simulink model "Design_of_an_Energy_Efficient_Hybrid_Electric_Vehicle"  (R2023a)
settings: Solver=FixedStepDiscrete  StartTime=0  StopTime=110  RelTol=1e-3  EnableMultiTasking=on
PreLoadFcn:
  | power_motordrive_IPMSM_FOC_data
InitFcn:
  | power_motordrive_IPMSM_FOC_data
  | Cdc  = 0.001;      % DC-link capacitor  [F]
  | AH0  = 280;        % Initial battery charge [hr*A]
  | Tmax=410;
  | 
  | %% Vehicle Parameters for Vehicle Dynamics 2
  | vehicle_mass = 2111;
  | wheel_radius = 0.228;
  | area =2.22;
  | drag_coefficient = 0.23;
  | air_density = 1.204;
  | gravity = 9.81;
  | rolling_res_ratio = 0.02;
  | 
  | % Differential drive parameters
  | gear_ratio = 5;
  | i_t   = gear_ratio ;
  | Rw=wheel_radius;
  | 
  | 
  | %% Sliding Mode Observer
  | pmsm.N_max=wmax;
  | pmsm.p=p
  | pmsm.Ld=Ld;
  | pmsm.Lq=Lq;
  | pmsm.Rs=Rs;
  | PU_System.V_base=(Vdc_nom/sqrt(3));
  | PU_System.I_base=lambda/(Lq-Ld);
  | max_torque=400
  | force_max_pedal=500
  | braking_torque_to_pedal_force_ratio=-4
undefined symbols (not defined in the file): BlkSampleTime, CurrentObserverGain, dataType, DiscIntNeverNeededParam, Fsw, gcbh, Ki_Ireg, Ki_wreg, Kp_Ireg, Kp_wreg, L_smo_gain, lambda, Ld, Limit_Ireg, Limit_wreg, Lq, MaxApplicationSpeed, MaxStatorCurrent, MaxStatorVoltage, NumBits1, NumBits2, p, Pmsm, PolePairs, QPLL, rpm_data, Sensorless, sigbuilder_block, SlidingLimit, Slope1, Slope2, sps_rtmsupport, StatorInductance, StatorResistance, Tmax_data, Tnom, Ts, Vdc_nom, wmax
libraries: fl_lib x27, nesl_utility x24, simulink x23, mcbcontrolslib x15, fl_ps_legacy_lib x9, spsStairGeneratorLib x7, sdl_lib x6, ee_lib x4, mcbpositiondecoderlib x4, BoomBox x3, tiiqmathlib x2, autolibshared x2
(part 3 of 4)

== system Design_of_an_Energy_Efficient_Hybrid_Electric_Vehicle/FOC/Speed Regulator1/PI regulator with anti-windup D1 ==
  note: Anti-windup mechanism: Method of conditionnal integration
      |
      | The integration is suspended if saturation occurs and the
      | control error is of the same sign as the control signal.
      |
      | [1] L.Rundqwist, "Anti-Reset Windup for PID Controllers," Ph.D. Thesis TRFT-1033,
      | Departement of Automatic Control, Lund Institute of Technology, Lund, Sweeden, 1991.
  Error : Inport  SampleTime=Ts
  Compare To Zero : simulink/Logic and Bit Operations/Compare To Zero  relop=>  OutDataTypeStr=uint8  ZeroCross=off
  Compare To Zero1 : simulink/Logic and Bit Operations/Compare To Zero  relop=<  OutDataTypeStr=uint8  ZeroCross=off
  Constant : Constant  Value=0
  Constant1 : Constant  Value=UpperLimit
  Constant3 : Constant  Value=LowerLimit
  Discrete-Time Integrator : DiscreteIntegrator  IntegratorMethod=Integration: Trapezoidal  InitialCondition=Init  SampleTime=Ts  LimitOutput=on  UpperSaturationLimit=UpperLimit  LowerSaturationLimit=LowerLimit  ShowStatePort=on  ICPrevOutput=DiscIntNeverNeededParam  ICPrevScaledInput=DiscIntNeverNeededParam
  Kp4 : Gain  Gain=Kp  SaturateOnIntegerOverflow=on  SampleTime=Ts  OutDataTypeStr=Inherit: Same as input  ParamDataTypeStr=Inherit: Same as input
  Kp5 : Gain  Gain=Ki  SaturateOnIntegerOverflow=on  SampleTime=Ts  OutDataTypeStr=Inherit: Same as input  ParamDataTypeStr=Inherit: Same as input
  Logical Operator : Logic  AllPortsSameDT=off  OutDataTypeStr=boolean
  Logical Operator1 : Logic  AllPortsSameDT=off  OutDataTypeStr=boolean
  Logical Operator2 : Logic  Operator=OR  AllPortsSameDT=off  OutDataTypeStr=boolean
  Relational Operator : RelationalOperator  OutDataTypeStr=boolean  InputSameDT=off
  Relational Operator1 : RelationalOperator  Operator=<=  OutDataTypeStr=boolean  InputSameDT=off
  Saturation2 : Saturate  UpperLimit=UpperLimit  LowerLimit=LowerLimit  SampleTime=Ts
  Sum1 : Sum  InputSameDT=on  SaturateOnIntegerOverflow=on  SampleTime=Ts  OutDataTypeStr=Inherit: Same as first input
  Sum6 : Sum  InputSameDT=on  SaturateOnIntegerOverflow=on  SampleTime=Ts  OutDataTypeStr=Inherit: Same as first input
  Switch : Switch  Criteria=u2 > Threshold  SaturateOnIntegerOverflow=off  InputSameDT=off
  Zero-Order Hold : ZeroOrderHold  SampleTime=Ts
  Out : Outport  SampleTime=Ts  InitialOutput=0
  wires:
  Constant/1 -> Switch/1
  Zero-Order Hold/1 -> Sum1/2, Sum6/1
  Discrete-Time Integrator/State -> Sum1/1
  Sum1/1 -> Relational Operator1/1, Relational Operator/1
  Logical Operator2/1 -> Switch/2
  Relational Operator/1 -> Logical Operator/1  "UpperLimit_is_Reached"
  Relational Operator1/1 -> Logical Operator1/1  "LowerLimit_Is_Reached"
  Constant1/1 -> Relational Operator/2
  Constant3/1 -> Relational Operator1/2
  Compare To Zero/1 -> Logical Operator/2  "Error_is_positive"
  Logical Operator/1 -> Logical Operator2/1
  Logical Operator1/1 -> Logical Operator2/2
  Compare To Zero1/1 -> Logical Operator1/2  "Error_is_negative"
  Error/1 -> Compare To Zero1/1, Compare To Zero/1, Kp4/1, Kp5/1
  Sum6/1 -> Saturation2/1
  Kp4/1 -> Zero-Order Hold/1
  Discrete-Time Integrator/1 -> Sum6/2
  Saturation2/1 -> Out/1
  Switch/1 -> Discrete-Time Integrator/1
  Kp5/1 -> Switch/3

== system Design_of_an_Energy_Efficient_Hybrid_Electric_Vehicle/FOC/Speed Regulator1/PI regulator with anti-windup D2 ==
  note: Anti-windup mechanism: Method of conditionnal integration
      |
      | The integration is suspended if saturation occurs and the
      | control error is of the same sign as the control signal.
      |
      | [1] L.Rundqwist, "Anti-Reset Windup for PID Controllers," Ph.D. Thesis TRFT-1033,
      | Departement of Automatic Control, Lund Institute of Technology, Lund, Sweeden, 1991.
  Error : Inport  SampleTime=Ts
  Compare To Zero : simulink/Logic and Bit Operations/Compare To Zero  relop=>  OutDataTypeStr=uint8  ZeroCross=off
  Compare To Zero1 : simulink/Logic and Bit Operations/Compare To Zero  relop=<  OutDataTypeStr=uint8  ZeroCross=off
  Constant : Constant  Value=0
  Constant1 : Constant  Value=UpperLimit
  Constant3 : Constant  Value=LowerLimit
  Discrete-Time Integrator : DiscreteIntegrator  IntegratorMethod=Integration: Trapezoidal  InitialCondition=Init  SampleTime=Ts  LimitOutput=on  UpperSaturationLimit=UpperLimit  LowerSaturationLimit=LowerLimit  ShowStatePort=on  ICPrevOutput=DiscIntNeverNeededParam  ICPrevScaledInput=DiscIntNeverNeededParam
  Kp4 : Gain  Gain=Kp  SaturateOnIntegerOverflow=on  SampleTime=Ts  OutDataTypeStr=Inherit: Same as input  ParamDataTypeStr=Inherit: Same as input
  Kp5 : Gain  Gain=Ki  SaturateOnIntegerOverflow=on  SampleTime=Ts  OutDataTypeStr=Inherit: Same as input  ParamDataTypeStr=Inherit: Same as input
  Logical Operator : Logic  AllPortsSameDT=off  OutDataTypeStr=boolean
  Logical Operator1 : Logic  AllPortsSameDT=off  OutDataTypeStr=boolean
  Logical Operator2 : Logic  Operator=OR  AllPortsSameDT=off  OutDataTypeStr=boolean
  Relational Operator : RelationalOperator  OutDataTypeStr=boolean  InputSameDT=off
  Relational Operator1 : RelationalOperator  Operator=<=  OutDataTypeStr=boolean  InputSameDT=off
  Saturation2 : Saturate  UpperLimit=UpperLimit  LowerLimit=LowerLimit  SampleTime=Ts
  Sum1 : Sum  InputSameDT=on  SaturateOnIntegerOverflow=on  SampleTime=Ts  OutDataTypeStr=Inherit: Same as first input
  Sum6 : Sum  InputSameDT=on  SaturateOnIntegerOverflow=on  SampleTime=Ts  OutDataTypeStr=Inherit: Same as first input
  Switch : Switch  Criteria=u2 > Threshold  SaturateOnIntegerOverflow=off  InputSameDT=off
  Zero-Order Hold : ZeroOrderHold  SampleTime=Ts
  Out : Outport  SampleTime=Ts  InitialOutput=0
  wires:
  Kp5/1 -> Switch/3
  Switch/1 -> Discrete-Time Integrator/1
  Saturation2/1 -> Out/1
  Discrete-Time Integrator/1 -> Sum6/2
  Kp4/1 -> Zero-Order Hold/1
  Sum6/1 -> Saturation2/1
  Error/1 -> Kp5/1, Kp4/1, Compare To Zero/1, Compare To Zero1/1
  Compare To Zero1/1 -> Logical Operator1/2  "Error_is_negative"
  Logical Operator1/1 -> Logical Operator2/2
  Logical Operator/1 -> Logical Operator2/1
  Compare To Zero/1 -> Logical Operator/2  "Error_is_positive"
  Constant3/1 -> Relational Operator1/2
  Constant1/1 -> Relational Operator/2
  Relational Operator1/1 -> Logical Operator1/1  "LowerLimit_Is_Reached"
  Relational Operator/1 -> Logical Operator/1  "UpperLimit_is_Reached"
  Logical Operator2/1 -> Switch/2
  Sum1/1 -> Relational Operator/1, Relational Operator1/1
  Discrete-Time Integrator/State -> Sum1/1
  Zero-Order Hold/1 -> Sum6/1, Sum1/2
  Constant/1 -> Switch/1

== system Design_of_an_Energy_Efficient_Hybrid_Electric_Vehicle/FOC/Speed Regulator1/VdVq Limiter ==
  VdVq_unsat : Inport
  Complex to Magnitude-Angle1 : ComplexToMagnitudeAngle
  Complex to Real-Imag : ComplexToRealImag
  Demux : Demux  Outputs=2
  Hypot : Math  Operator=hypot
  Magnitude-Angle to Complex : MagnitudeAngleToComplex
  Mux : Mux  Inputs=2
  Real-Imag to Complex : RealImagToComplex
  Saturation1 : Saturate  UpperLimit=2/sqrt(3)  LowerLimit=0
  VdVq : Outport
  ModIndex : Outport  Port=2
  wires:
  Real-Imag to Complex/1 -> Complex to Magnitude-Angle1/1
  Saturation1/1 -> Magnitude-Angle to Complex/1
  Complex to Magnitude-Angle1/2 -> Magnitude-Angle to Complex/2
  Complex to Magnitude-Angle1/1 -> Saturation1/1
  Magnitude-Angle to Complex/1 -> Complex to Real-Imag/1
  Demux/1 -> Real-Imag to Complex/1
  Demux/2 -> Real-Imag to Complex/2
  VdVq_unsat/1 -> Demux/1
  Complex to Real-Imag/1 -> Hypot/1, Mux/1
  Complex to Real-Imag/2 -> Hypot/2, Mux/2
  Mux/1 -> VdVq/1
  Hypot/1 -> ModIndex/1

== system Design_of_an_Energy_Efficient_Hybrid_Electric_Vehicle/Test_Sequences/Test_Sequence/IDC ==
  Demux : Demux  Tag=STV Demux  Outputs=1
      settings: DisplayOption=none
  FromWs : FromWorkspace  Tag=STV FromWs  VariableName=tuvar  SampleTime=Ts
      SigBuilderData=|
      | common.afterFinalStr = 'Extrapolate'
      | common.sampleTime = 'Ts'
      | dataSet.timeRange = [0 130]
      | dataSet.name = 'Test 1'
      | sbobj.Groups.Name = 'Test 1'
      | sbobj.Groups.Signals.Name = 'Speed'
      | sbobj.Groups.Signals.XData = [0 17 20 28 30 35 40 50 55 60 75 80 90 120 130]
      | sbobj.Groups.Signals.YData = [0 0 17.5 6 6 30 24 24 41 35.5 35.5 31 40 5 -8.4]
      | sbobj.Groups.TimeRange = [0 130]
  Speed : Outport  Tag=STV Outport  VectorParamsAs1DForOutWhenUnconnected=off
  wires:
  FromWs/1 -> Demux/1
  Demux/1 -> Speed/1

== system Design_of_an_Energy_Efficient_Hybrid_Electric_Vehicle/Test_Sequences/Test_Sequence/Load_Torque ==
  Demux : Demux  Tag=STV Demux  Outputs=1
      settings: DisplayOption=none
  FromWs : FromWorkspace  Tag=STV FromWs  VariableName=tuvar
      SigBuilderData=|
      | common.afterFinalStr = 'Extrapolate'
      | common.sampleTime = '0'
      | dataSet.timeRange = [0 14]
      | dataSet.name = 'Test 1'
      | sbobj.Groups.Name = 'Test 1'
      | sbobj.Groups.Signals.Name = 'Signal 2'
      | sbobj.Groups.Signals.XData = [0 4 5 5 14]
      | sbobj.Groups.Signals.YData = [0.945 0.945 0.945 0.3 0.3]
      | sbobj.Groups.TimeRange = [0 14]
  Signal 2 : Outport  Tag=STV Outport
  wires:
  FromWs/1 -> Demux/1
  Demux/1 -> Signal 2/1

== system Design_of_an_Energy_Efficient_Hybrid_Electric_Vehicle/Test_Sequences/Test_Sequence/Ref_Speed ==
  Demux : Demux  Tag=STV Demux  Outputs=1
      settings: DisplayOption=none
  FromWs : FromWorkspace  Tag=STV FromWs  VariableName=tuvar
      SigBuilderData=|
      | common.afterFinalStr = 'Extrapolate'
      | common.sampleTime = '0'
      | dataSet.timeRange = [0 13]
      | dataSet.name = 'Test 1'
      | sbobj.Groups.Name = 'Test 1'
      | sbobj.Groups.Signals.Name = 'Speed'
      | sbobj.Groups.Signals.XData = [0 0.65 1.3 2 4 6 7.5 9.3 12 13]
      | sbobj.Groups.Signals.YData = [0 0 0.2 0.2 1 1 1.5 1.5 0 0]
      | sbobj.Groups.TimeRange = [0 13]
  Speed : Outport  Tag=STV Outport  VectorParamsAs1DForOutWhenUnconnected=off
  wires:
  FromWs/1 -> Demux/1
  Demux/1 -> Speed/1

== system Design_of_an_Energy_Efficient_Hybrid_Electric_Vehicle/FOC/Speed Regulator1/Calculate position and speed/Sliding Mode Observer ==
  InputSignals : Inport
  Data Type Conversion : DataTypeConversion  OutDataTypeStr=boolean  SaturateOnIntegerOverflow=off  RndMeth=Floor
  Demux1 : Demux
  EEMF Model : Subsystem
  Logical Operator : Logic  Operator=NOT  IconShape=distinctive  AllPortsSameDT=off  OutDataTypeStr=boolean
  Mux : Mux  Inputs=2
  Scope : Scope  NumInputPorts=2
  Scope1 : Scope  NumInputPorts=4
  Sliding Mode Observer : Subsystem  Commented=on  mask(Sliding Mode Observer){CurrentObserverGain=.1, SlidingLimit=3, PositionUnit=Per unit, PositionDataType=dataType, SpeedUnit=Per unit, PerUnitSpeed=PU_System.N_base, SpeedDataType=dataType, BlkSampleTime=Ts, StatorResistance=pmsm.Rs, StatorInductance=pmsm.Ld, MaxApplicationSpeed=pmsm.N_max, PolePairs=pmsm.p, MaxStatorVoltage=PU_System.V_base, MaxStatorCurrent=PU_System.I_base}
      mask prompts: CurrentObserverGain "Current observer gain:"; SlidingLimit "Sliding surface limit:"; PositionUnit "Position unit:"; PositionDataType "Position datatype:"; SpeedUnit "Speed unit"; PerUnitSpeed "Per unit speed (RPM):"; SpeedDataType "Speed datatype:"; BlkSampleTime "Block sample time (S):"; StatorResistance "Stator resistance (ohm):"; StatorInductance "Stator inductance (H):"; MaxApplicationSpeed "Maximum application speed (RPM):"; PolePairs "Number of pole pairs:"; MaxStatorVoltage "Per unit reference stator voltage:"; MaxStatorCurrent "Per unit reference stator current:"
      mask help:
      | <p>Compute &#952;<sub>e</sub> (electrical position) and &#969;<sub>m</sub> (mechanical speed) of a PMSM from the measured per unit voltage and current in the stationary reference frame.
      | <br><br>
      | Use the Current observer gain and Sliding surface limit parameters to tune Sliding Mode Observer (SMO). To improve stability, increase the Sliding surface limit or reduce Current observer gain. To reduce distortion, increase the Current observer gain.
      | <br><br>
      | Enter the peak-to-peak line-to-line voltage and peak-to-peak line current of the stator, in the Per unit reference parameters. Ensure that the values for Per Unit reference stator voltage, Per unit reference stator current, and Maximum application speed conform to the maximum applicable limits for the SMO.</P>
      mask init:
      | mcb.internal.SMOCb('MaskInitFcn',gcbh);
      mask Help: eval('mcb.internal.helpview(''slidingmodeobserver'')')
      mask TypeOptions PositionUnit: Degrees | Radians | Per unit
      mask TypeOptions SpeedUnit: Degrees/sec | Radians/sec | RPM | Per unit
      mask Callback SpeedUnit: mcb.internal.SMOCb('SpeedUnit',gcbh);
      mask DialogControl Container4 Prompt: Observer Parameters
      mask DialogControl Container7 Prompt: Motor Parameters
      mask Display:
      | color('black');
      | port_label('input',1, 'V_{\alpha}', 'interpreter', 'tex');
      | port_label('input',2, 'V_{\beta}', 'interpreter', 'tex');
      | port_label('input',3, 'I_{\alpha}', 'interpreter', 'tex');
      | port_label('input',4, 'I_{\beta}', 'interpreter', 'tex');
      | port_label('input',5, 'Rst', 'interpreter', 'tex');
      | port_label('output',1, '\theta_{e}', 'interpreter', 'tex');
      | port_label('output',2, '\omega_{m}', 'interpreter', 'tex');
      | fprintf('SMO');
  Step : Step  SampleTime=0
  Subsystem : Subsystem  Commented=on
  Position/Speed : Outport
  wires:
  Mux/1 -> Position/Speed/1
  Demux1/1 -> EEMF Model/1(Valpha), Scope1/1
  Demux1/2 -> EEMF Model/2(Vbeta), Scope1/2
  Demux1/4 -> EEMF Model/4(Ibeta), Scope1/4  "Ibeta"
  Demux1/3 -> EEMF Model/3(Ialpha), Scope1/3  "Ialpha"
  EEMF Model/1(Theta) -> Scope/1, Mux/1
  EEMF Model/2(Speed) -> Scope/2, Mux/2
  InputSignals/1 -> Demux1/1
  Step/1 -> Data Type Conversion/1
  Logical Operator/1 -> EEMF Model/5(Reset)
  Data Type Conversion/1 -> Logical Operator/1

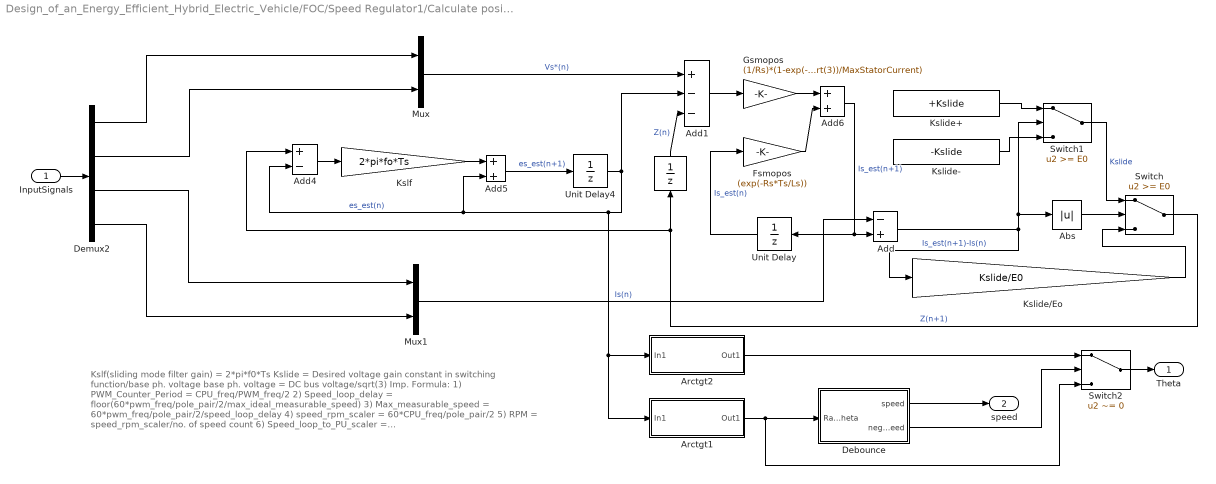
== system Design_of_an_Energy_Efficient_Hybrid_Electric_Vehicle/FOC/Speed Regulator1/Calculate position and speed/Sliding Mode Observer (SMO) ==
  note: Kslf(sliding mode filter gain) = 2*pi*f0*Ts
      | Kslide = Desired voltage gain constant in switching function/base ph. voltage
      | base ph. voltage = DC bus voltage/sqrt(3)
      |
      | Imp. Formula:
      |
      | 1) PWM_Counter_Period = CPU_freq/PWM_freq/2
      | 2) Speed_loop_delay = floor(60*pwm_freq/pole_pair/2/max_ideal_measurable_speed)
      | 3) Max_measurable_speed = 60*pwm_freq/pole_pair/2/speed_loop_delay
      | 4) speed_rpm_scaler = 60*CPU_freq/pole_pair/2
      | 5) RPM = speed_rpm_scaler/no. of speed count
      | 6) Speed_loop_to_PU_scaler = Max_measurable_speed/Speed_per_unit_scaler
      |
      | 7) Fsmopos = exp(-motor.rs/motor.ls/PWM_frequency)
      | 8)Gsmopos = motor.base_voltage/motor.base_current/motor.rs*(1-Fsmopos)
      | 9)motor.base_voltage = 38.29; % Base peak phase voltage (volt), maximum measurable DC Bus(66.32V)/sqrt(3)
      | 10)motor.base_current = 8.6; % Base peak phase current (amp) , maximum measurable peak current
      | 11)motor.base_freq = 200; % Base electrical frequency (Hz)
  InputSignals : Inport
  " " : UnitDelay  SampleTime=-1  HasFrameUpgradeWarning=on
  Abs : Abs  SaturateOnIntegerOverflow=off
  Add : Sum  Inputs=-+  OutDataTypeStr=Inherit: Same as first input
  Add1 : Sum  Inputs=+--  OutDataTypeStr=Inherit: Inherit via back propagation
  Add4 : Sum  Inputs=+-  OutDataTypeStr=Inherit: Same as first input
  Add5 : Sum  OutDataTypeStr=Inherit: Same as first input
  Add6 : Sum  OutDataTypeStr=Inherit: Same as first input
  Arctgt1 : Subsystem
  Arctgt2 : Subsystem
  Debounce : Subsystem
  Demux2 : Demux
  Fsmopos : Gain  Gain=(exp(-Rs*Ts/Ls))  OutDataTypeStr=Inherit: Same as input  ParamDataTypeStr=Inherit: Same as input
  Gsmopos : Gain  Gain=(1/Rs)*(1-exp(-Rs*Ts/Ls)*(MaxStatorVoltage/sqrt(3))/MaxStatorCurrent)  OutDataTypeStr=Inherit: Same as input  ParamDataTypeStr=Inherit: Same as input
  Kslf : Gain  Gain=2*pi*fo*Ts  OutDataTypeStr=Inherit: Same as input  ParamDataTypeStr=Inherit: Same as input
  Kslide+ : Constant  Value=+Kslide  OutDataTypeStr=fixdt(1,32,17)
  Kslide- : Constant  Value=-Kslide  OutDataTypeStr=fixdt(1,32,17)
  Kslide/Eo : Gain  Gain=Kslide/E0  OutDataTypeStr=Inherit: Same as input  ParamDataTypeStr=Inherit: Same as input
  Mux : Mux  Inputs=2
  Mux1 : Mux  Inputs=2
  Switch : Switch  Threshold=E0  OutDataTypeStr=Inherit: Inherit via back propagation  SaturateOnIntegerOverflow=off  InputSameDT=off
  Switch1 : Switch  Threshold=E0  OutDataTypeStr=Inherit: Inherit via back propagation  SaturateOnIntegerOverflow=off  InputSameDT=off
  Switch2 : Switch  Criteria=u2 ~= 0  SaturateOnIntegerOverflow=off  InputSameDT=off
  Unit Delay : UnitDelay  SampleTime=-1  HasFrameUpgradeWarning=on
  Unit Delay4 : UnitDelay  SampleTime=-1  HasFrameUpgradeWarning=on
  Theta : Outport  VectorParamsAs1DForOutWhenUnconnected=off
  speed : Outport  Port=2  VectorParamsAs1DForOutWhenUnconnected=off
  wires:
  Unit Delay/1 -> Fsmopos/1  "Is_est(n)"
  " "/1 -> Add1/3  "Z(n)"
  Add/1 -> Kslide/Eo/1, Abs/1, Switch1/2  "Is_est(n+1)-Is(n)"
  Add1/1 -> Gsmopos/1
  Demux2/2 -> Mux/2
  Mux/1 -> Add1/1  "Vs*(n)"
  Add4/1 -> Kslf/1
  Unit Delay4/1 -> Arctgt2/1(In1), Arctgt1/1(In1), Add5/2, Add4/2, Add1/2  "es_est(n)"
  Kslf/1 -> Add5/1
  Add5/1 -> Unit Delay4/1  "es_est(n+1)"
  Gsmopos/1 -> Add6/1
  Fsmopos/1 -> Add6/2
  Add6/1 -> Add/2, Unit Delay/1  "Is_est(n+1)"
  Demux2/3 -> Mux1/1
  Demux2/4 -> Mux1/2
  Abs/1 -> Switch/2
  Kslide/Eo/1 -> Switch/3
  Switch1/1 -> Switch/1  "Kslide"
  Kslide+/1 -> Switch1/1
  Kslide-/1 -> Switch1/3
  Switch/1 -> Add4/1, " "/1  "Z(n+1)"
  Mux1/1 -> Add/1  "Is(n)"
  Arctgt1/1(Out1) -> Switch2/3, Debounce/1(Raw_theta)
  Arctgt2/1(Out1) -> Switch2/1
  Switch2/1 -> Theta/1
  Debounce/1(speed) -> speed/1
  Debounce/2(negative speed) -> Switch2/2
  InputSignals/1 -> Demux2/1
  Demux2/1 -> Mux/1

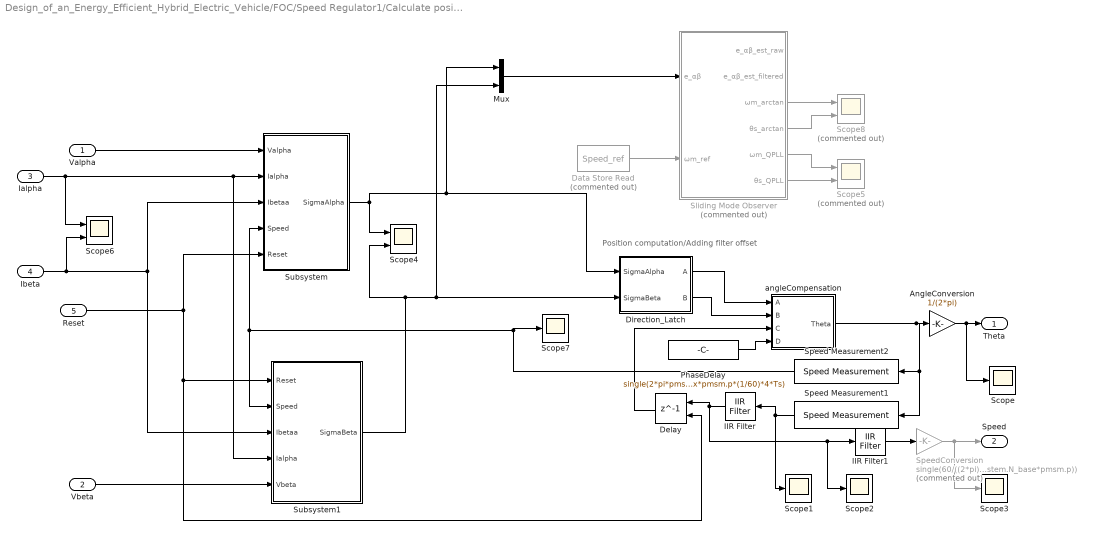
== system Design_of_an_Energy_Efficient_Hybrid_Electric_Vehicle/FOC/Speed Regulator1/Calculate position and speed/Sliding Mode Observer/EEMF Model ==
  note: Position computation/Adding filter offset
  Valpha : Inport
  Vbeta : Inport  Port=2
  Ialpha : Inport  Port=3
  Ibeta : Inport  Port=4
  Reset : Inport  Port=5
  AngleConversion : Gain  Gain=1/(2*pi)  OutDataTypeStr=single
  Data Store Read : DataStoreRead  Commented=on  DataStoreName=Speed_ref  IndexOptions=Index vector (dialog)  Indices=1  OutputSizes=1
  Delay : Delay  DelayLength=1  ExternalReset=Level
      settings: InputPortMap=u0,r5
  Direction_Latch : Subsystem
  IIR Filter : mcbcontrolslib/IIR Filter  VariantControl=Low Pass Filter  VariantSelect=Low-pass  Filter_constant=single(Ts*pmsm.N_max*pmsm.p/120)  advancedSettings=off  Ts=50e-6  cutOff_freq=12.7835
  IIR Filter1 : mcbcontrolslib/IIR Filter  VariantControl=Low Pass Filter  VariantSelect=Low-pass  Filter_constant=single(Ts*pmsm.N_max*pmsm.p/120)  advancedSettings=off  Ts=50e-6  cutOff_freq=12.7835
  Mux : Mux  Inputs=2
  PhaseDelay : Constant  Value=single(2*pi*pmsm.N_max*pmsm.p*(1/60)*4*Ts)  OutDataTypeStr=Inherit: Inherit via back propagation  SampleTime=-1
  Scope{,1..3,7} (5 alike) : Scope
  Scope4 : Scope  NumInputPorts=2
  Scope5 : Scope  Commented=on  NumInputPorts=2
  Scope6 : Scope  NumInputPorts=2
  Scope8 : Scope  Commented=on  NumInputPorts=2
  Sliding Mode Observer : Subsystem  Commented=on
  Speed Measurement1 : mcbpositiondecoderlib/Speed Measurement  PositionUnit=Radians  PositionScalingDatatype=uint32  SpeedCalculationMode=Maximum application speed  SampleTimeAsync=Ts  MaximumApplicationSpeed=pmsm.N_max*pmsm.p  SpeedResolution=5e-6  DelayLength=61  MaximumMeasurableSpeed=24193.5484  MeasurableSpeedResolution=1.1266e-05  SpeedUnit=Radians/Sec  PerUnitSpeed=1000  SpeedDataType=single
  Speed Measurement2 : mcbpositiondecoderlib/Speed Measurement  PositionUnit=Radians  PositionScalingDatatype=uint32  SpeedCalculationMode=Maximum application speed  SampleTimeAsync=Ts  MaximumApplicationSpeed=pmsm.N_max*pmsm.p  SpeedResolution=5e-6  DelayLength=61  MaximumMeasurableSpeed=24193.5484  MeasurableSpeedResolution=1.1266e-05  SpeedUnit=Per unit based on maximum measurable speed  PerUnitSpeed=1000  SpeedDataType=single
  SpeedConversion : Gain  Commented=on  Gain=single(60/((2*pi)*PU_System.N_base*pmsm.p))  OutDataTypeStr=single
  Subsystem : Subsystem
  Subsystem1 : Subsystem
  angleCompensation : Subsystem  TreatAsAtomicUnit=on
  Theta : Outport  VectorParamsAs1DForOutWhenUnconnected=off
  Speed : Outport  Port=2  VectorParamsAs1DForOutWhenUnconnected=off
  wires:
  Reset/1 -> Subsystem/5(Reset), Delay/2, Subsystem1/1(Reset)
  SpeedConversion/1 -> Scope3/1, Speed/1
  Ibeta/1 -> Scope6/2, Subsystem1/3(Ibetaa), Subsystem/3(Ibetaa)
  Vbeta/1 -> Subsystem1/5(Vbeta)
  PhaseDelay/1 -> angleCompensation/4(D)
  Valpha/1 -> Subsystem/1(Valpha)
  angleCompensation/1(Theta) -> Speed Measurement2/1, Speed Measurement1/1, AngleConversion/1
  Speed Measurement1/1 -> Scope1/1, IIR Filter/1
  AngleConversion/1 -> Scope/1, Theta/1
  Direction_Latch/1(A) -> angleCompensation/1(A)
  Ialpha/1 -> Scope6/1, Subsystem1/4(Ialpha), Subsystem/2(Ialpha)
  Direction_Latch/2(B) -> angleCompensation/2(B)
  Delay/1 -> angleCompensation/3(C)
  Subsystem/1(SigmaAlpha) -> Mux/1, Direction_Latch/1(SigmaAlpha), Scope4/1
  Subsystem1/1(SigmaBeta) -> Mux/2, Direction_Latch/2(SigmaBeta), Scope4/2
  IIR Filter/1 -> IIR Filter1/1, Scope2/1, Delay/1
  Speed Measurement2/1 -> Scope7/1, Subsystem/4(Speed), Subsystem1/2(Speed)
  IIR Filter1/1 -> SpeedConversion/1
  Mux/1 -> Sliding Mode Observer/1(e_αβ)
  Data Store Read/1 -> Sliding Mode Observer/2(ωm_ref)
  Sliding Mode Observer/5(ωm_QPLL) -> Scope5/1
  Sliding Mode Observer/6(θs_QPLL) -> Scope5/2
  Sliding Mode Observer/3(ωm_arctan) -> Scope8/1
  Sliding Mode Observer/4(θs_arctan) -> Scope8/2

== system Design_of_an_Energy_Efficient_Hybrid_Electric_Vehicle/FOC/Speed Regulator1/Calculate position and speed/Sliding Mode Observer/Sliding Mode Observer ==
  note: Position computation/Adding filter offset
  Valpha : Inport
  Vbeta : Inport  Port=2
  Ialpha : Inport  Port=3
  Ibeta : Inport  Port=4
  Reset : Inport  Port=5
  AngleConversion : Gain  Gain=1/(2*pi)  OutDataTypeStr=PositionDataType
  Delay : Delay  DelayLength=1  ExternalReset=Level
      settings: InputPortMap=u0,r5
  Direction_Latch : Subsystem
  IIR Filter : mcbcontrolslib/IIR Filter  VariantControl=Low Pass Filter  VariantSelect=Low-pass  Filter_constant=single(BlkSampleTime(1)*MaxApplicationSpeed*PolePairs/120)  advancedSettings=off  Ts=50e-6
  PhaseDelay : Constant  Value=single((StatorResistance+(CurrentObserverGain/SlidingLimit))/StatorInductance)  OutDataTypeStr=Inherit: Inherit via back propagation
  Scope{,1..3} (4 alike) : Scope
  Speed Measurement : mcbpositiondecoderlib/Speed Measurement  PositionUnit=Radians  PositionScalingDatatype=uint32  SpeedCalculationMode=Maximum application speed  SampleTimeAsync=BlkSampleTime  MaximumApplicationSpeed=MaxApplicationSpeed*PolePairs  SpeedResolution=5e-6  DelayLength=14  MaximumMeasurableSpeed=40000  MeasurableSpeedResolution=1.8626e-05  SpeedUnit=Radians/Sec  PerUnitSpeed=1000  SpeedDataType=single
  SpeedConversion : Gain  Gain=single(60/((2*pi)*PerUnitSpeed*PolePairs))  OutDataTypeStr=SpeedDataType
  Subsystem : Subsystem
  Subsystem1 : Subsystem
  angleCompensation : Subsystem  TreatAsAtomicUnit=on
  Theta : Outport  VectorParamsAs1DForOutWhenUnconnected=off
  Speed : Outport  Port=2  VectorParamsAs1DForOutWhenUnconnected=off
  wires:
  Reset/1 -> Delay/2, Subsystem1/3(Reset), Subsystem/3(Reset)
  Subsystem1/1(SigmaBeta) -> Direction_Latch/2(SigmaBeta)
  Subsystem/1(SigmaAlpha) -> Direction_Latch/1(SigmaAlpha)
  Direction_Latch/2(B) -> angleCompensation/2(B)
  Direction_Latch/1(A) -> angleCompensation/1(A)
  AngleConversion/1 -> Theta/1
  Delay/1 -> angleCompensation/3(C)
  PhaseDelay/1 -> angleCompensation/4(D)
  angleCompensation/1(Theta) -> Speed Measurement/1, Scope/1, AngleConversion/1
  Ibeta/1 -> Subsystem1/2(Ibetaa)
  Ialpha/1 -> Subsystem/2(Ialpha)
  Vbeta/1 -> Subsystem1/1(Vbeta)
  Valpha/1 -> Subsystem/1(Valpha)
  Speed Measurement/1 -> Scope1/1, IIR Filter/1
  IIR Filter/1 -> Delay/1, SpeedConversion/1, Scope2/1
  SpeedConversion/1 -> Scope3/1, Speed/1

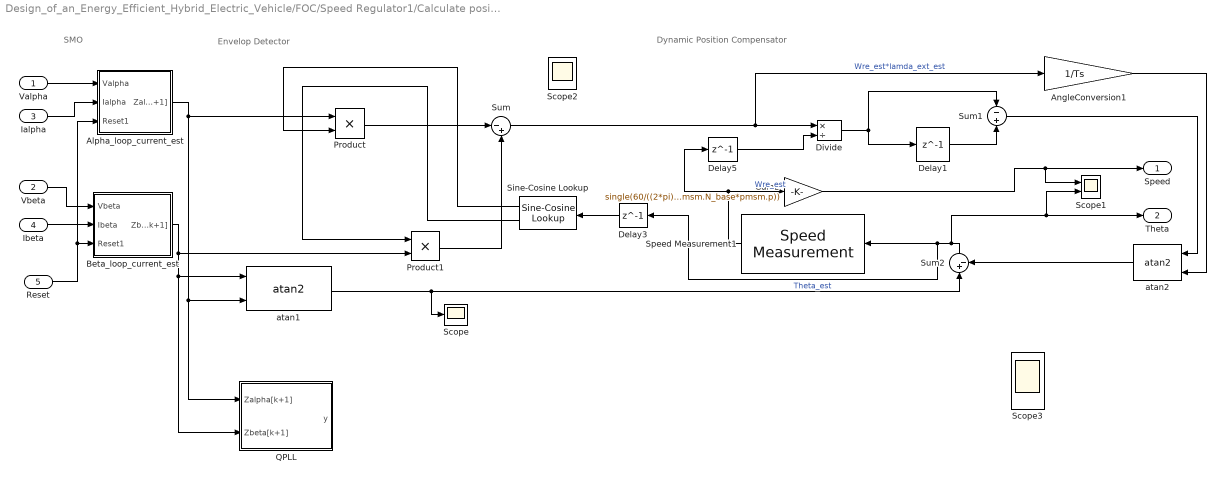
== system Design_of_an_Energy_Efficient_Hybrid_Electric_Vehicle/FOC/Speed Regulator1/Calculate position and speed/Sliding Mode Observer/Subsystem ==
  note: Dynamic Position Compensator
  note: Envelop Detector
  note: SMO
  Valpha : Inport
  Vbeta : Inport  Port=2
  Ialpha : Inport  Port=3
  Ibeta : Inport  Port=4
  Reset : Inport  Port=5
  Alpha_loop_current_est : Subsystem
  AngleConversion1 : Gain  Gain=1/Ts  OutDataTypeStr=single
  Beta_loop_current_est : Subsystem
  Delay1 : Delay  DelayLength=1
  Delay3 : Delay  DelayLength=1
  Delay5 : Delay  DelayLength=1
  Divide : Product  Inputs=*/  OutDataTypeStr=single
  Gain2 : Gain  Gain=single(60/((2*pi)*pmsm.N_base*pmsm.p))
  Product : Product
  Product1 : Product
  QPLL : Subsystem
  Scope : Scope
  Scope1 : Scope  NumInputPorts=2
  Scope2 : Scope  NumInputPorts=3
  Scope3 : Scope  NumInputPorts=3
  Sine-Cosine Lookup : mcbcontrolslib/Sine-Cosine Lookup  AngleInput=Per-unit  N_points=1024
  Speed Measurement1 : mcbpositiondecoderlib/Speed Measurement  PositionUnit=Per unit  PositionScalingDatatype=uint32  SpeedCalculationMode=Maximum application speed  SampleTimeAsync=Ts  MaximumApplicationSpeed=pmsm.N_max*pmsm.p  SpeedResolution=5e-6  DelayLength=14  MaximumMeasurableSpeed=40000  MeasurableSpeedResolution=1.8626e-05  SpeedUnit=Per unit based on maximum measurable speed  PerUnitSpeed=1000  SpeedDataType=single
  Sum : Sum  Inputs=|-+
  Sum1 : Sum  Inputs=-+
  Sum2 : Sum  Inputs=|+-
  atan1 : mcbcontrolslib/atan2  outputUnit=PerUnit
  atan2 : mcbcontrolslib/atan2  outputUnit=PerUnit
  Speed : Outport  VectorParamsAs1DForOutWhenUnconnected=off
  Theta : Outport  Port=2  VectorParamsAs1DForOutWhenUnconnected=off
  wires:
  Valpha/1 -> Alpha_loop_current_est/1(Valpha)
  Vbeta/1 -> Beta_loop_current_est/1(Vbeta)
  Ialpha/1 -> Alpha_loop_current_est/2(Ialpha)
  Ibeta/1 -> Beta_loop_current_est/2(Ibeta)
  Reset/1 -> Alpha_loop_current_est/3(Reset1), Beta_loop_current_est/3(Reset1)
  Sine-Cosine Lookup/1 -> Product/2
  Sine-Cosine Lookup/2 -> Product1/1
  Product/1 -> Sum/1
  Speed Measurement1/1 -> Delay5/1, Gain2/1  "Wre_est"
  Divide/1 -> Delay1/1, Sum1/1
  Delay1/1 -> Sum1/2
  Sum2/1 -> Scope1/2, Theta/1, Speed Measurement1/1, Delay3/1  "Theta_est"
  Gain2/1 -> Scope1/1, Speed/1
  Product1/1 -> Sum/2
  Sum/1 -> AngleConversion1/1, Divide/1  "Wre_est*lamda_ext_est"
  atan2/1 -> Sum2/2
  Sum1/1 -> atan2/1
  AngleConversion1/1 -> atan2/2
  atan1/1 -> Scope/1, Sum2/1
  Alpha_loop_current_est/1(Zalpha[k+1]) -> QPLL/1(Zalpha[k+1]), atan1/2, Product/1
  Delay3/1 -> Sine-Cosine Lookup/1
  Delay5/1 -> Divide/2
  Beta_loop_current_est/1(Zbeta[k+1]) -> QPLL/2(Zbeta[k+1]), atan1/1, Product1/2

== system Design_of_an_Energy_Efficient_Hybrid_Electric_Vehicle/FOC/Speed Regulator1/Calculate position and speed/Sliding Mode Observer (SMO)/Arctgt1 ==
  In1 : Inport
  Arctangent IQN : tiiqmathlib/Arctangent IQN  tanOption=atan2PU (per unit)
  Demux1 : Demux  Outputs=2
  Gain1 : Gain  Gain=-1  OutDataTypeStr=Inherit: Same as input  ParamDataTypeStr=Inherit: Same as input
  Out1 : Outport  VectorParamsAs1DForOutWhenUnconnected=off
  wires:
  In1/1 -> Demux1/1
  Arctangent IQN/1 -> Out1/1
  Demux1/1 -> Gain1/1
  Gain1/1 -> Arctangent IQN/2
  Demux1/2 -> Arctangent IQN/1

== system Design_of_an_Energy_Efficient_Hybrid_Electric_Vehicle/FOC/Speed Regulator1/Calculate position and speed/Sliding Mode Observer (SMO)/Arctgt2 ==
  In1 : Inport
  Arctangent IQN : tiiqmathlib/Arctangent IQN  tanOption=atan2PU (per unit)
  Demux1 : Demux  Outputs=2
  Gain1 : Gain  Gain=-1  OutDataTypeStr=Inherit: Same as input  ParamDataTypeStr=Inherit: Same as input
  Out1 : Outport  VectorParamsAs1DForOutWhenUnconnected=off
  wires:
  In1/1 -> Demux1/1
  Arctangent IQN/1 -> Out1/1
  Demux1/1 -> Arctangent IQN/2
  Demux1/2 -> Gain1/1
  Gain1/1 -> Arctangent IQN/1

== system Design_of_an_Energy_Efficient_Hybrid_Electric_Vehicle/FOC/Speed Regulator1/Calculate position and speed/Sliding Mode Observer (SMO)/Debounce ==
  Raw_theta : Inport
  Add : Sum  Inputs=+-  OutDataTypeStr=uint16
  Compare To Constant2 : simulink/Logic and Bit Operations/Compare To Constant  relop=<  const=32768+2000  OutDataTypeStr=boolean
  Compare To Constant3 : simulink/Logic and Bit Operations/Compare To Constant  relop=>  const=32768-2000  OutDataTypeStr=boolean
  Constant : Constant  Value=0  OutDataTypeStr=fixdt(1,32,17)
  Data Type Conversion1 : DataTypeConversion  OutDataTypeStr=fixdt(1,32,15)  ConvertRealWorld=Stored Integer (SI)  SaturateOnIntegerOverflow=off  RndMeth=Floor
  Data Type Conversion2 : DataTypeConversion  OutDataTypeStr=int16  ConvertRealWorld=Stored Integer (SI)  SaturateOnIntegerOverflow=off  RndMeth=Floor
  Data Type Conversion3 : DataTypeConversion  OutDataTypeStr=fixdt(1,32,16)  SaturateOnIntegerOverflow=off  RndMeth=Floor
  Data Type Conversion4 : DataTypeConversion  OutDataTypeStr=uint16  ConvertRealWorld=Stored Integer (SI)  SaturateOnIntegerOverflow=off  RndMeth=Floor
  Logical Operator1 : Logic  AllPortsSameDT=off  OutDataTypeStr=boolean
  Relay : Relay  OnSwitchValue=0.05  OffSwitchValue=-0.05  OnOutputValue=0  OffOutputValue=1
  Speed IIR filter : Subsystem
  Speed Loop Delay : Delay  DelayLength=SMO_params6
  Speed_loop_to_PU_scaler : Gain  Gain=SMO_params7  ParamDataTypeStr=fixdt(1,32,17)  OutDataTypeStr=fixdt(1,32,17)
  Switch : Switch  Criteria=u2 ~= 0  SaturateOnIntegerOverflow=off  InputSameDT=off
  speed : Outport  VectorParamsAs1DForOutWhenUnconnected=off
  negative speed : Outport  Port=2  VectorParamsAs1DForOutWhenUnconnected=off
  wires:
  Add/1 -> Compare To Constant3/1, Compare To Constant2/1, Data Type Conversion2/1
  Raw_theta/1 -> Data Type Conversion3/1
  Speed Loop Delay/1 -> Add/2
  Data Type Conversion2/1 -> Data Type Conversion1/1
  Data Type Conversion3/1 -> Data Type Conversion4/1
  Data Type Conversion1/1 -> Speed_loop_to_PU_scaler/1
  Data Type Conversion4/1 -> Add/1, Speed Loop Delay/1
  Compare To Constant2/1 -> Logical Operator1/1
  Compare To Constant3/1 -> Logical Operator1/2
  Logical Operator1/1 -> Switch/2
  Constant/1 -> Switch/1
  Switch/1 -> Speed IIR filter/1(Speed)
  Speed_loop_to_PU_scaler/1 -> Switch/3
  Relay/1 -> negative speed/1
  Speed IIR filter/1(Filtered speed) -> speed/1, Relay/1

== system Design_of_an_Energy_Efficient_Hybrid_Electric_Vehicle/FOC/Speed Regulator1/Calculate position and speed/Sliding Mode Observer/EEMF Model/Direction_Latch ==
  SigmaAlpha : Inport
  SigmaBeta : Inport  Port=2
  Compare To Zero : simulink/Logic and Bit Operations/Compare To Zero  relop=>  OutDataTypeStr=boolean
  Compare To Zero1 : simulink/Logic and Bit Operations/Compare To Zero  relop=>  OutDataTypeStr=boolean
  Dir_Sense : Subsystem  TreatAsAtomicUnit=on
  If : If
  Merge : Merge
  Merge1 : Merge
  Subsystem2 : Subsystem
  Subsystem3 : Subsystem
  A : Outport
  B : Outport  Port=2
  wires:
  Dir_Sense/1(Sign) -> If/1
  Compare To Zero/1 -> Dir_Sense/1(A), Dir_Sense/Trigger
  Compare To Zero1/1 -> Dir_Sense/2(B)
  Merge/1 -> A/1
  Merge1/1 -> B/1
  Subsystem2/2(Out2) -> Merge1/1
  Subsystem3/1(Out2) -> Merge1/2
  If/2 -> Subsystem3/Action
  Subsystem3/2(Out1) -> Merge/2
  Subsystem2/1(Out1) -> Merge/1
  If/1 -> Subsystem2/Action
  SigmaBeta/1 -> Compare To Zero1/1, Subsystem2/2(SigmaBeta), Subsystem3/1(SigmaBeta)
  SigmaAlpha/1 -> Subsystem3/2(SigmaAlpha), Subsystem2/1(SigmaAlpha), Compare To Zero/1

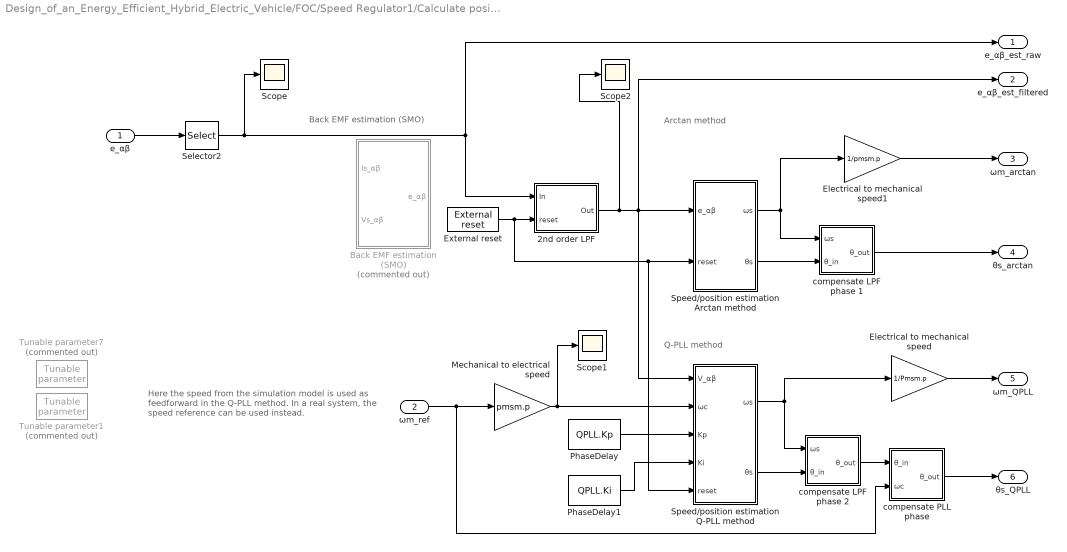
== system Design_of_an_Energy_Efficient_Hybrid_Electric_Vehicle/FOC/Speed Regulator1/Calculate position and speed/Sliding Mode Observer/EEMF Model/Sliding Mode Observer ==
  note: Q-PLL method
  note: Arctan method
  note: Back EMF estimation (SMO)
  note: Here the speed from the simulation model is used as
      | feedforward in the Q-PLL method. In a real system, the
      | speed reference can be used instead.
  e_αβ : Inport
  ωm_ref : Inport  Port=2
  2nd order LPF : Subsystem  mask{fc=Sensorless.fc_EMF}
      mask prompts: fc "Cut-off frequency [Hz]"
      mask help: Second-order infinite-impulse-response low-pass filter.
      mask init:
      | tc = 1/fc;
  Back EMF estimation (SMO) : Subsystem  Commented=on  mask{Rs=Pmsm.Rs, Ls=Pmsm.Ls, a=Sensorless.a, Ks=Sensorless.Ks}
      mask prompts: Rs "Stator resistance Rs"; Ls "Stator inductance Ls"; a "Sigmoid "a" parameter"; Ks "SMO gain Ks"
  Electrical to mechanical speed : Gain  Gain=1/Pmsm.p
  Electrical to mechanical speed1 : Gain  Gain=1/pmsm.p
  External reset : BoomBox/External reset  KBID=kb0504
  Mechanical to electrical speed : Gain  Gain=pmsm.p  ParamDataTypeStr=single
  PhaseDelay : Constant  Value=QPLL.Kp  OutDataTypeStr=single  SampleTime=-1
  PhaseDelay1 : Constant  Value=QPLL.Ki  OutDataTypeStr=single  SampleTime=-1
  Scope : Scope
  Scope1 : Scope
  Scope2 : Scope
  Selector2 : Selector  InputPortWidth=2  IndexOptions=Index vector (dialog)  Indices=[1 2]  OutputSizes=1
  Speed/position estimation Arctan method : Subsystem
  Speed/position estimation Q-PLL method : Subsystem
  Tunable parameter1 : BoomBox/Tunable parameter  Commented=on  VARNAME=Ki_QPLL  INITIALVAL=QPLL.Ki  DATA_TYPE=single  CAN_ENABLED=off  CAN_ADDRESS=0  can_endianness=Little-endian  init_baudrate=0  CAN_BAUDRATE=1000000  ETH_ENABLED=off  ETH_PORT=2000  eth_endianness=Little-endian  SIM_OUT=Initial value  STEP_TIMES=[0.1 0.2]  STEP_DATA=[1 2]  KBID=kb0501  CAN_BIG_ENDIAN=0  ETH_BIG_ENDIAN=0  CAN_MB_ID=0  ETH_MB_ID=1
  Tunable parameter7 : BoomBox/Tunable parameter  Commented=on  VARNAME=Kp_QPLL  INITIALVAL=QPLL.Kp  DATA_TYPE=single  CAN_ENABLED=off  CAN_ADDRESS=0  can_endianness=Little-endian  init_baudrate=0  CAN_BAUDRATE=1000000  ETH_ENABLED=off  ETH_PORT=2000  eth_endianness=Little-endian  SIM_OUT=Initial value  STEP_TIMES=[0.1 0.2]  STEP_DATA=[1 2]  KBID=kb0501  CAN_BIG_ENDIAN=0  ETH_BIG_ENDIAN=0  CAN_MB_ID=0  ETH_MB_ID=1
  compensate LPF phase 1 : Subsystem  mask{fc=Sensorless.fc_EMF}
      mask prompts: fc "Cut-off frequency of the LPF [Hz]"
      mask help: Compensates the phase-shift induced by a 2nd order low-pass filter.
      mask init:
      | wc = 2*pi*fc;
  compensate LPF phase 2 : Subsystem  mask{fc=Sensorless.fc_EMF}
      mask prompts: fc "Cut-off frequency of the LPF [Hz]"
      mask help: Compensates the phase-shift induced by a 2nd order low-pass filter.
      mask init:
      | wc = 2*pi*fc;
  compensate PLL phase : Subsystem
  e_αβ_est_raw : Outport
  e_αβ_est_filtered : Outport  Port=2
  ωm_arctan : Outport  Port=3
  θs_arctan : Outport  Port=4
  ωm_QPLL : Outport  Port=5
  θs_QPLL : Outport  Port=6
  wires:
  Selector2/1 -> Scope/1, e_αβ_est_raw/1, 2nd order LPF/1(In)
  PhaseDelay/1 -> Speed/position estimation Q-PLL method/3(Kp)
  PhaseDelay1/1 -> Speed/position estimation Q-PLL method/4(Ki)
  2nd order LPF/1(Out) -> Scope2/1, e_αβ_est_filtered/1, Speed/position estimation Arctan method/1(e_αβ), Speed/position estimation Q-PLL method/1(V_αβ)
  Mechanical to electrical speed/1 -> Scope1/1, Speed/position estimation Q-PLL method/2(ωc)
  ωm_ref/1 -> compensate PLL phase/2(ωc), Mechanical to electrical speed/1
  Electrical to mechanical speed1/1 -> ωm_arctan/1
  Speed/position estimation Arctan method/1(ωs) -> Electrical to mechanical speed1/1, compensate LPF phase 1/1(ωs)
  Electrical to mechanical speed/1 -> ωm_QPLL/1
  Speed/position estimation Q-PLL method/2(θs) -> compensate LPF phase 2/2(θ_in)
  Speed/position estimation Arctan method/2(θs) -> compensate LPF phase 1/2(θ_in)
  compensate LPF phase 2/1(θ_out) -> compensate PLL phase/1(θ_in)
  compensate PLL phase/1(θ_out) -> θs_QPLL/1
  External reset/1 -> Speed/position estimation Q-PLL method/5(reset), Speed/position estimation Arctan method/2(reset), 2nd order LPF/2(reset)
  compensate LPF phase 1/1(θ_out) -> θs_arctan/1
  e_αβ/1 -> Selector2/1
  Speed/position estimation Q-PLL method/1(ωs) -> Electrical to mechanical speed/1, compensate LPF phase 2/1(ωs)

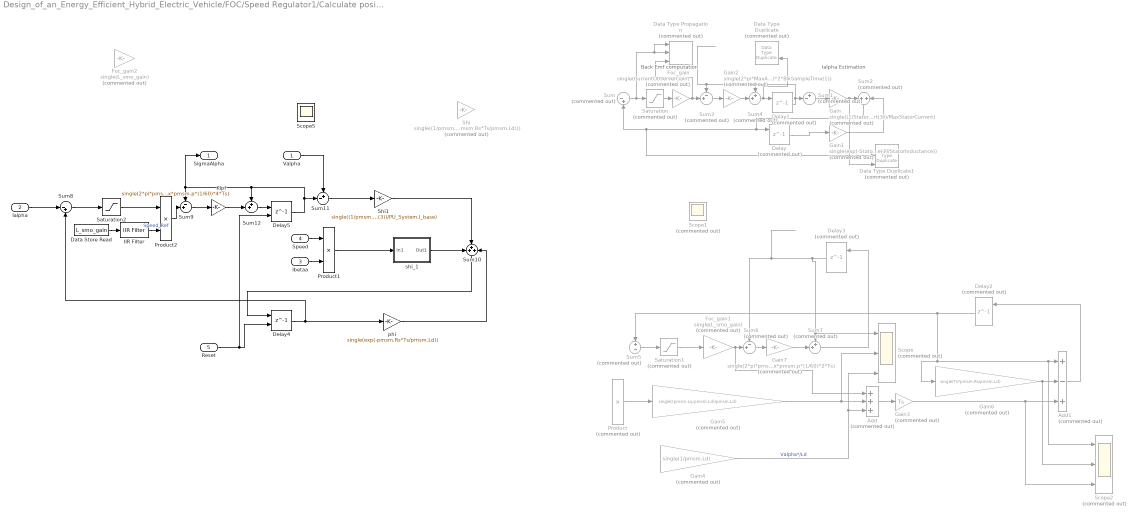
== system Design_of_an_Energy_Efficient_Hybrid_Electric_Vehicle/FOC/Speed Regulator1/Calculate position and speed/Sliding Mode Observer/EEMF Model/Subsystem ==
  note: Back Emf computation
  note: Ialpha Estimation
  Valpha : Inport
  Ialpha : Inport  Port=2
  Ibetaa : Inport  Port=3
  Speed : Inport  Port=4
  Reset : Inport  Port=5
  Add : Sum  Commented=on  Inputs=+++
  Add1 : Sum  Commented=on  Inputs=+-+
  Data Store Read : DataStoreRead  DataStoreName=L_smo_gain  IndexOptions=Index vector (dialog)  Indices=1  OutputSizes=1
  Data Type Duplicate : DataTypeDuplicate  Commented=on
  Data Type Duplicate1 : DataTypeDuplicate  Commented=on  NumInputPorts=3
  Data Type Propagation : simulink/Signal Attributes/Data Type Propagation  Commented=on  PropDataType=fixdt(1, 16)  IfRefDouble=double  IfRefSingle=single  IsSigned=IsSigned1 or IsSigned2  NumBitsBase=max([NumBits1 NumBits2])  NumBitsMult=1  NumBitsAdd=0  NumBitsAllowFinal=1:128  PropScalingMode=Obtain via best precision  PropScaling=2^-10  ValuesUsedBestPrec=[SlidingLimit*CurrentObserverGain -SlidingLimit*CurrentObserverGain]  SlopeBase=min([Slope1 Slope2])  SlopeMult=1  SlopeAdd=0  BiasBase=Bias1  BiasMult=1  BiasAdd=0
  Delay{,1..3} (4 alike) : Delay  Commented=on  DelayLength=1  ExternalReset=Level
      settings: InputPortMap=u0,r5
  Delay4 : Delay  DelayLength=1  ExternalReset=Level
      settings: InputPortMap=u0,r5
  Delay5 : Delay  DelayLength=1  ExternalReset=Level
      settings: InputPortMap=u0,r5
  Foc_gain : Gain  Commented=on  Gain=single(CurrentObserverGain)  OutDataTypeStr=Inherit: Inherit via back propagation
  Foc_gain1 : Gain  Commented=on  Gain=single(L_smo_gain)  OutDataTypeStr=Inherit: Inherit via back propagation
  Foc_gain2 : Gain  Commented=on  Gain=single(L_smo_gain)  OutDataTypeStr=Inherit: Inherit via back propagation
  Gain : Gain  Commented=on  Gain=single((1/StatorResistance)*(1-exp(-StatorResistance*BlkSampleTime(1)/StatorInductance))*(MaxStatorVoltage/sqrt(3))/MaxStatorCurrent)  OutDataTypeStr=Inherit: Same as input
  Gain1 : Gain  Commented=on  Gain=single(exp(-StatorResistance*BlkSampleTime(1)/StatorInductance))  OutDataTypeStr=Inherit: Same as input
  Gain2 : Gain  Commented=on  Gain=single(2*pi*MaxApplicationSpeed*PolePairs*(1/60)*2*BlkSampleTime(1))  OutDataTypeStr=Inherit: Same as input
  Gain3 : Gain  Commented=on  Gain=Ts
  Gain4 : Gain  Commented=on  Gain=single(1/pmsm.Ld)
  Gain5 : Gain  Commented=on  Gain=single((pmsm.Lq-pmsm.Ld)/pmsm.Ld)
  Gain6 : Gain  Commented=on  Gain=single(Ts*pmsm.Rs/pmsm.Ld)
  Gain7 : Gain  Commented=on  Gain=single(2*pi*pmsm.N_max*pmsm.p*(1/60)*2*Ts)  OutDataTypeStr=Inherit: Same as input
  IIR Filter : mcbcontrolslib/IIR Filter  VariantControl=Low Pass Filter  VariantSelect=Low-pass  Filter_constant=1  advancedSettings=off  Ts=50e-6  cutOff_freq=Inf
  Klpf : Gain  Gain=single(2*pi*pmsm.N_max*pmsm.p*(1/60)*4*Ts)  OutDataTypeStr=Inherit: Same as input
  Product : Product  Commented=on
  Product1 : Product
  Product2 : Product
  Saturation : Saturate  Commented=on  UpperLimit=SlidingLimit  LowerLimit=-1*SlidingLimit
  Saturation1 : Saturate  Commented=on  UpperLimit=SlidingLimit  LowerLimit=-1*SlidingLimit
  Saturation2 : Saturate  UpperLimit=SlidingLimit  LowerLimit=-1*SlidingLimit
  Scope : Scope  Commented=on  NumInputPorts=3
  Scope1 : Scope  Commented=on  NumInputPorts=2
  Scope2 : Scope  Commented=on  NumInputPorts=3
  Scope5 : Scope
  Shi : Gain  Commented=on  Gain=single((1/pmsm.Rs)*(1-exp(-pmsm.Rs*Ts/pmsm.Ld)))  OutDataTypeStr=Inherit: Same as input
  Shi1 : Gain  Gain=single((1/pmsm.Rs)*(1-exp(-pmsm.Rs*Ts/pmsm.Ld))*(PU_System.V_base/sqrt(3))/PU_System.I_base)  OutDataTypeStr=Inherit: Same as input
  Sum : Sum  Commented=on  Inputs=|-+  OutDataTypeStr=Inherit: Same as first input
  Sum1 : Sum  Commented=on  Inputs=+-|  OutDataTypeStr=Inherit: Same as first input
  Sum10 : Sum  Inputs=+++  OutDataTypeStr=Inherit: Same as first input
  Sum11 : Sum  Inputs=+-|  OutDataTypeStr=Inherit: Same as first input
  Sum12 : Sum  Inputs=++|  OutDataTypeStr=Inherit: Inherit via back propagation
  Sum2 : Sum  Commented=on  OutDataTypeStr=Inherit: Same as first input
  Sum3 : Sum  Commented=on  Inputs=-+|  OutDataTypeStr=Inherit: Same as first input
  Sum4 : Sum  Commented=on  Inputs=++|  OutDataTypeStr=Inherit: Inherit via back propagation
  Sum5 : Sum  Commented=on  Inputs=+-  OutDataTypeStr=Inherit: Same as first input
  Sum6 : Sum  Commented=on  Inputs=-+|  OutDataTypeStr=Inherit: Same as first input
  Sum7 : Sum  Commented=on  Inputs=++|  OutDataTypeStr=Inherit: Inherit via back propagation
  Sum8 : Sum  Inputs=|-+  OutDataTypeStr=Inherit: Same as first input
  Sum9 : Sum  Inputs=-+|  OutDataTypeStr=Inherit: Same as first input
  phi : Gain  Gain=single(exp(-pmsm.Rs*Ts/pmsm.Ld))  OutDataTypeStr=Inherit: Same as input
  shi_1 : Subsystem
  SigmaAlpha : Outport  VectorParamsAs1DForOutWhenUnconnected=off
  wires:
  ? -> Delay/2, Delay1/2
  Sum/1 -> Saturation/1, Data Type Propagation/2, Data Type Propagation/1
  ? -> Sum/1, Data Type Duplicate1/1
  ? -> Sum1/1, Data Type Duplicate/1
  Gain1/1 -> Sum2/2
  Gain/1 -> Sum2/1, Data Type Duplicate1/3
  Sum1/1 -> Gain/1
  Delay/1 -> Gain1/1
  Sum4/1 -> Delay1/1, Data Type Duplicate/2
  Sum2/1 -> Delay/1, Sum/2, Data Type Duplicate1/2
  Delay1/1 -> Sum1/2, Sum3/1, Sum4/1
  Saturation/1 -> Foc_gain/1
  Foc_gain/1 -> Data Type Propagation/3, Sum3/2
  Sum3/1 -> Gain2/1
  Gain2/1 -> Sum4/2
  ? -> Sum5/2, Scope1/1
  Sum5/1 -> Saturation1/1
  Saturation1/1 -> Foc_gain1/1
  ? -> Product/1
  ? -> Product/2
  Product/1 -> Gain5/1
  ? -> Gain4/1
  Gain5/1 -> Scope/2, Add/2
  Gain4/1 -> Scope/3, Add/3  "Valpha*/Ld"
  Add/1 -> Gain3/1
  Delay2/1 -> Sum5/1, Gain6/1, Scope2/1, Add1/1
  Gain3/1 -> Scope2/3, Add1/3
  Gain6/1 -> Scope2/2, Add1/2
  Add1/1 -> Delay2/1
  ? -> Delay3/2, Delay2/2
  Delay3/1 -> Scope/1, Sum7/1, Sum6/1
  Foc_gain1/1 -> Add/1, Sum6/2
  Sum6/1 -> Gain7/1
  Gain7/1 -> Sum7/2
  Sum7/1 -> Delay3/1
  Ialpha/1 -> Sum8/1
  Sum8/1 -> Saturation2/1
  Saturation2/1 -> Product2/1
  Product2/1 -> Sum9/2
  Delay4/1 -> phi/1, Sum8/2
  Speed/1 -> Product1/1
  Ibetaa/1 -> Product1/2
  Product1/1 -> shi_1/1(In1)
  shi_1/1(Out1) -> Sum10/1
  Sum11/1 -> Shi1/1
  phi/1 -> Sum10/3
  Sum10/1 -> Delay4/1
  Valpha/1 -> Sum11/1
  Sum9/1 -> Klpf/1
  Klpf/1 -> Sum12/2
  Sum12/1 -> Delay5/1
  Delay5/1 -> Sum11/2, SigmaAlpha/1, Sum9/1, Sum12/1
  Reset/1 -> Delay5/2, Delay4/2
  Shi1/1 -> Sum10/2
  Data Store Read/1 -> IIR Filter/1
  IIR Filter/1 -> Product2/2  "Speed_Ref"

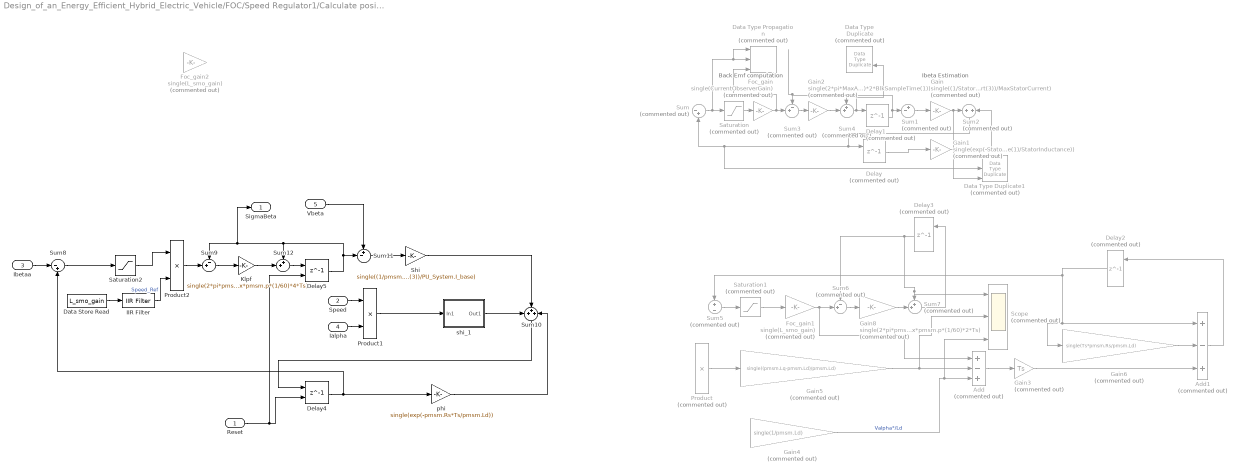
== system Design_of_an_Energy_Efficient_Hybrid_Electric_Vehicle/FOC/Speed Regulator1/Calculate position and speed/Sliding Mode Observer/EEMF Model/Subsystem1 ==
  note: Back Emf computation
  note: Ibeta Estimation
  Reset : Inport
  Speed : Inport  Port=2
  Ibetaa : Inport  Port=3
  Ialpha : Inport  Port=4
  Vbeta : Inport  Port=5
  Add : Sum  Commented=on  Inputs=+-+
  Add1 : Sum  Commented=on  Inputs=+-+
  Data Store Read : DataStoreRead  DataStoreName=L_smo_gain  IndexOptions=Index vector (dialog)  Indices=1  OutputSizes=1
  Data Type Duplicate : DataTypeDuplicate  Commented=on
  Data Type Duplicate1 : DataTypeDuplicate  Commented=on  NumInputPorts=3
  Data Type Propagation : simulink/Signal Attributes/Data Type Propagation  Commented=on  PropDataType=fixdt(1, 16)  IfRefDouble=double  IfRefSingle=single  IsSigned=IsSigned1 or IsSigned2  NumBitsBase=max([NumBits1 NumBits2])  NumBitsMult=1  NumBitsAdd=0  NumBitsAllowFinal=1:128  PropScalingMode=Obtain via best precision  PropScaling=2^-10  ValuesUsedBestPrec=[SlidingLimit*CurrentObserverGain -SlidingLimit*CurrentObserverGain]  SlopeBase=min([Slope1 Slope2])  SlopeMult=1  SlopeAdd=0  BiasBase=Bias1  BiasMult=1  BiasAdd=0
  Delay{,1..3} (4 alike) : Delay  Commented=on  DelayLength=1  ExternalReset=Level
      settings: InputPortMap=u0,r5
  Delay4 : Delay  DelayLength=1  ExternalReset=Level
      settings: InputPortMap=u0,r5
  Delay5 : Delay  DelayLength=1  ExternalReset=Level
      settings: InputPortMap=u0,r5
  Foc_gain : Gain  Commented=on  Gain=single(CurrentObserverGain)  OutDataTypeStr=Inherit: Inherit via back propagation
  Foc_gain1 : Gain  Commented=on  Gain=single(L_smo_gain)  OutDataTypeStr=Inherit: Inherit via back propagation
  Foc_gain2 : Gain  Commented=on  Gain=single(L_smo_gain)  OutDataTypeStr=Inherit: Inherit via back propagation
  Gain : Gain  Commented=on  Gain=single((1/StatorResistance)*(1-exp(-StatorResistance*BlkSampleTime(1)/StatorInductance))*(MaxStatorVoltage/sqrt(3))/MaxStatorCurrent)  OutDataTypeStr=Inherit: Same as input
  Gain1 : Gain  Commented=on  Gain=single(exp(-StatorResistance*BlkSampleTime(1)/StatorInductance))  OutDataTypeStr=Inherit: Same as input
  Gain2 : Gain  Commented=on  Gain=single(2*pi*MaxApplicationSpeed*PolePairs*(1/60)*2*BlkSampleTime(1))  OutDataTypeStr=Inherit: Same as input
  Gain3 : Gain  Commented=on  Gain=Ts
  Gain4 : Gain  Commented=on  Gain=single(1/pmsm.Ld)
  Gain5 : Gain  Commented=on  Gain=single((pmsm.Lq-pmsm.Ld)/pmsm.Ld)
  Gain6 : Gain  Commented=on  Gain=single(Ts*pmsm.Rs/pmsm.Ld)
  Gain8 : Gain  Commented=on  Gain=single(2*pi*pmsm.N_max*pmsm.p*(1/60)*2*Ts)  OutDataTypeStr=Inherit: Same as input
  IIR Filter : mcbcontrolslib/IIR Filter  VariantControl=Low Pass Filter  VariantSelect=Low-pass  Filter_constant=1  advancedSettings=off  Ts=50e-6  cutOff_freq=Inf
  Klpf : Gain  Gain=single(2*pi*pmsm.N_max*pmsm.p*(1/60)*4*Ts)  OutDataTypeStr=Inherit: Same as input
  Product : Product  Commented=on
  Product1 : Product
  Product2 : Product
  Saturation : Saturate  Commented=on  UpperLimit=SlidingLimit  LowerLimit=-1*SlidingLimit
  Saturation1 : Saturate  Commented=on  UpperLimit=SlidingLimit  LowerLimit=-1*SlidingLimit
  Saturation2 : Saturate  UpperLimit=SlidingLimit  LowerLimit=-1*SlidingLimit
  Scope : Scope  Commented=on  NumInputPorts=3
  Shi : Gain  Gain=single((1/pmsm.Rs)*(1-exp(-pmsm.Rs*Ts/pmsm.Ld))*(PU_System.V_base/sqrt(3))/PU_System.I_base)  OutDataTypeStr=Inherit: Same as input
  Sum : Sum  Commented=on  Inputs=|-+  OutDataTypeStr=Inherit: Same as first input
  Sum1 : Sum  Commented=on  Inputs=+-|  OutDataTypeStr=Inherit: Same as first input
  Sum10 : Sum  Inputs=+++  OutDataTypeStr=Inherit: Same as first input
  Sum11 : Sum  Inputs=+-|  OutDataTypeStr=Inherit: Same as first input
  Sum12 : Sum  Inputs=++|  OutDataTypeStr=Inherit: Inherit via back propagation
  Sum2 : Sum  Commented=on  OutDataTypeStr=Inherit: Same as first input
  Sum3 : Sum  Commented=on  Inputs=-+|  OutDataTypeStr=Inherit: Same as first input
  Sum4 : Sum  Commented=on  Inputs=++|  OutDataTypeStr=Inherit: Inherit via back propagation
  Sum5 : Sum  Commented=on  Inputs=+-  OutDataTypeStr=Inherit: Same as first input
  Sum6 : Sum  Commented=on  Inputs=-+|  OutDataTypeStr=Inherit: Same as first input
  Sum7 : Sum  Commented=on  Inputs=++|  OutDataTypeStr=Inherit: Inherit via back propagation
  Sum8 : Sum  Inputs=|-+  OutDataTypeStr=Inherit: Same as first input
  Sum9 : Sum  Inputs=-+|  OutDataTypeStr=Inherit: Same as first input
  phi : Gain  Gain=single(exp(-pmsm.Rs*Ts/pmsm.Ld))  OutDataTypeStr=Inherit: Same as input
  shi_1 : Subsystem
  SigmaBeta : Outport  VectorParamsAs1DForOutWhenUnconnected=off
  wires:
  ? -> Delay1/2, Delay/2
  Sum/1 -> Saturation/1, Data Type Propagation/2, Data Type Propagation/1
  ? -> Sum/1, Data Type Duplicate1/1
  ? -> Sum1/1, Data Type Duplicate/1
  Gain1/1 -> Sum2/2
  Saturation/1 -> Foc_gain/1
  Gain/1 -> Sum2/1, Data Type Duplicate1/3
  Sum1/1 -> Gain/1
  Foc_gain/1 -> Sum3/2, Data Type Propagation/3
  Delay/1 -> Gain1/1
  Sum4/1 -> Delay1/1, Data Type Duplicate/2
  Sum2/1 -> Delay/1, Sum/2, Data Type Duplicate1/2
  Delay1/1 -> Sum1/2, Sum3/1, Sum4/1
  Sum3/1 -> Gain2/1
  Gain2/1 -> Sum4/2
  Sum5/1 -> Saturation1/1
  Gain3/1 -> Add1/3
  Add/1 -> Gain3/1
  ? -> Sum5/2
  Gain4/1 -> Scope/3, Add/3  "Valpha*/Ld"
  ? -> Delay3/2, Delay2/2
  Gain5/1 -> Scope/2, Add/2
  Product/1 -> Gain5/1
  ? -> Gain4/1
  Gain6/1 -> Add1/2
  Saturation1/1 -> Foc_gain1/1
  Add1/1 -> Delay2/1
  Delay2/1 -> Sum5/1, Gain6/1, Add1/1
  ? -> Product/2
  ? -> Product/1
  Delay3/1 -> Sum6/1, Scope/1, Sum7/1
  Gain8/1 -> Sum7/2
  Sum6/1 -> Gain8/1
  Foc_gain1/1 -> Add/1, Sum6/2
  Sum7/1 -> Delay3/1
  Reset/1 -> Delay5/2, Delay4/2
  Product2/1 -> Sum9/2
  Ibetaa/1 -> Sum8/1
  Delay5/1 -> Sum11/2, SigmaBeta/1, Sum9/1, Sum12/1
  Ialpha/1 -> Product1/2
  Sum9/1 -> Klpf/1
  Vbeta/1 -> Sum11/1
  phi/1 -> Sum10/3
  Sum11/1 -> Shi/1
  Sum12/1 -> Delay5/1
  Sum10/1 -> Delay4/1
  Speed/1 -> Product1/1
  shi_1/1(Out1) -> Sum10/1
  Saturation2/1 -> Product2/1
  Product1/1 -> shi_1/1(In1)
  Sum8/1 -> Saturation2/1
  Klpf/1 -> Sum12/2
  Shi/1 -> Sum10/2
  Delay4/1 -> phi/1, Sum8/2
  Data Store Read/1 -> IIR Filter/1
  IIR Filter/1 -> Product2/2  "Speed_Ref"
